simulink model "Temperaturregelung"  (R2021a)
settings: Solver=VariableStepAuto  StartTime=0.0  StopTime=10.0  RelTol=1e-3
undefined symbols (not defined in the file): sigbuilder_block
settings Model: Creator=Oceaner  LastModifiedBy=Oceaner

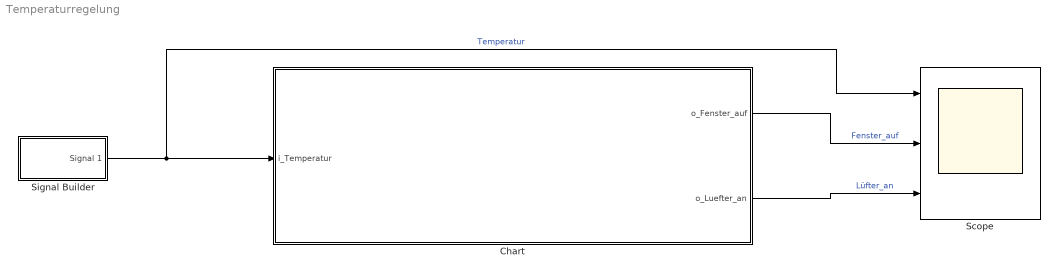
== system Temperaturregelung ==
  Chart : Stateflow chart  TreatAsAtomicUnit=on
  Scope : Scope  NumInputPorts=3
  Signal Builder : Subsystem  Tag=STV Subsys  LoadFcn=sigbuilder_block('load');  StartFcn=sigbuilder_block('start');  StopFcn=sigbuilder_block('stop');  ClipboardFcn=sigbuilder_block('clipboard');  mask(Sigbuilder block){tuvar=[0:10]}
      mask help: Simulink:masks:SigbuilderBlock_MD
      mask init:
      | if ~strcmp(get_param(bdroot(gcbh),'SimulationStatus'),'stopped') tuvar = sigbuilder_block('maskInit'); end
      settings: CopyFcn=sigbuilder_block('copy');  DeleteFcn=sigbuilder_block('delete');  ModelCloseFcn=sigbuilder_block('modelClose');  PreSaveFcn=sigbuilder_block('preSave');  PauseFcn=sigbuilder_block('pause');  ContinueFcn=sigbuilder_block('continue');  NameChangeFcn=sigbuilder_block('namechange');  OpenFcn=sigbuilder_block('open',[437.6 199.2 550.4 400 ]);  CloseFcn=sigbuilder_block('close');
      mask Display: plot(0, 0, 100, 100,[2, 2, 32, 32, 2], [68, 8, 8, 68, 68],[32, 2], [38, 38], [32, 19, 2],[53, 60, 44], [32, 17, 17, 2],[16, 16, 31, 31]);txt = getActiveGroup(gcbh);text(2, 100, txt,'verticalAlignment', 'top');
  wires:
  Signal Builder/1(Signal 1) -> Chart/1(i_Temperatur), Scope/1  "Temperatur"
  Chart/1(o_Fenster_auf) -> Scope/2  "Fenster_auf"
  Chart/2(o_Luefter_an) -> Scope/3  "Lüfter_an"

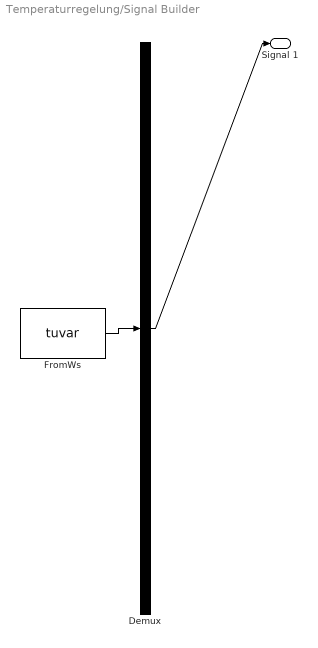
== system Temperaturregelung/Signal Builder ==
  Demux : Demux  Tag=STV Demux  Outputs=1
      settings: DisplayOption=none
  FromWs : FromWorkspace  Tag=STV FromWs  VariableName=tuvar
      SigBuilderData=|
      | common.afterFinalStr = 'Extrapolate'
      | common.sampleTime = 0
      | dataSet.timeRange = [0 10]
      | dataSet.name = 'Group 1'
      | sbobj.Groups.Name = 'Group 1'
      | sbobj.Groups.Signals.Name = 'Signal 1'
      | sbobj.Groups.Signals.XData = [0 0.05 1.85 2.65 3.3 4.6 4.6 5.3 5.95 5.95 6.6 6.6 7.8 8.35 10]
      | sbobj.Groups.Signals.YData = [1 1 47.5 10.5 23.5 1 40 25 57.5 70.5 47.5 1 37.5 16.5 1]
  Signal 1 : Outport  Tag=STV Outport
  wires:
  FromWs/1 -> Demux/1
  Demux/1 -> Signal 1/1

== stateflow chart Temperaturregelung/Chart ==
  state Luefter [parallel]
    settings: executionOrder=1
    state o_Luefter_aus1
      en:o_Luefter_an=0;
    state o_Luefter_an1
      en:o_Luefter_an=1;
    (default) -> o_Luefter_aus1
    o_Luefter_aus1 -> o_Luefter_an1 : [i_Temperatur>30]
    o_Luefter_an1 -> o_Luefter_aus1 : [i_Temperatur<25]
  state Fenster [parallel]
    settings: executionOrder=2
    state o_Fenster_zu1
      en:o_Fenster_auf=0
    state o_Fenster_auf1
      en:o_Fenster_auf=1;
    (default) -> o_Fenster_zu1
    o_Fenster_zu1 -> o_Fenster_auf1 : [i_Temperatur>25]
    o_Fenster_auf1 -> o_Fenster_zu1 : [i_Temperatur<20]
  data: o_Fenster_auf output; i_Temperatur input; o_Luefter_an output
